simulink library "DriveSpeed"  (R2024a)
settings: Solver=VariableStepAuto  StartTime=0.0  StopTime=10.0  RelTol=1e-3
undefined symbols (not defined in the file or in its folder): GearRatio, WheelRadius
settings Model: Creator=hyuga  LastModifiedBy=hyuga
settings ConfigComp: CovBoundaryAbsTol=1.0e-5

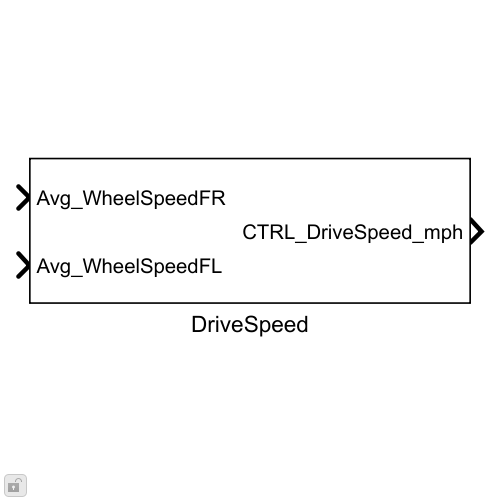
[thumbnail: Simulink's stored preview of the top-level diagram]
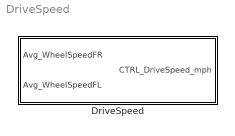
== system DriveSpeed ==
  DriveSpeed : Subsystem

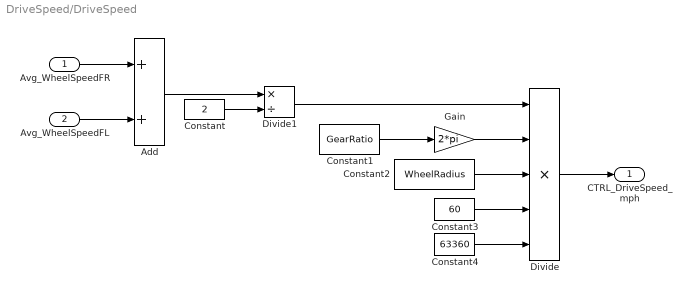
== system DriveSpeed/DriveSpeed ==
  Avg_WheelSpeedFR : Inport
  Avg_WheelSpeedFL : Inport  Port=2
  Add : Sum
  Constant : Constant  Value=2
  Constant1 : Constant  Value=GearRatio
  Constant2 : Constant  Value=WheelRadius
  Constant3 : Constant  Value=60
  Constant4 : Constant  Value=63360
  Divide : Product  Inputs=*****
  Divide1 : Product  Inputs=*/
  Gain : Gain  Gain=2*pi
  CTRL_DriveSpeed_mph : Outport
  wires:
  Divide1/1 -> Divide/1
  Constant/1 -> Divide1/2
  Add/1 -> Divide1/1
  Divide/1 -> CTRL_DriveSpeed_mph/1
  Constant4/1 -> Divide/5
  Constant3/1 -> Divide/4
  Constant2/1 -> Divide/3
  Gain/1 -> Divide/2
  Constant1/1 -> Gain/1
  Avg_WheelSpeedFL/1 -> Add/2
  Avg_WheelSpeedFR/1 -> Add/1
